simulink model "RflysimIndoorController_r2018b_N6_V8"  (R2018b)
settings: Solver=ode4  StartTime=0.0  StopTime=inf  FixedStep=ts  MaxStep=0.6  RelTol=1e-3
values from neighbouring files (symbols this model uses):
  l_v = 5    [RflyMain.m]    (also in RflyMain_N12_V6.m; RflyMain_N6_V3.m; RflyMain_N6_V4.m; RflyMain_V2.m)
  p_target = [200,10]    [RflyMain.m]    (also in RflyMain_N12_V6.m; RflyMain_N6_V3.m; RflyMain_N6_V4.m; RflyMain_V2.m)
  ra = 0.6    [RflyMain.m]    (also in RflyMain_N12_V6.m; RflyMain_N6_V3.m; RflyMain_N6_V4.m; RflyMain_V2.m)
  rs = 0.25    [RflyMain.m]    (also in RflyMain_N12_V6.m; RflyMain_N6_V3.m; RflyMain_N6_V4.m; RflyMain_V2.m)
  rt1 = 0.25    [RflyMain_N6_V4.m]
  rt2 = 1.5    [RflyMain_N6_V4.m]
  ts = [0 0]    [QuadModel2D.m]    (also in RflyMain.m = 0.01; RflyMain_N12_V6.m = 0.05; RflyMain_N6_V3.m = 0.05; RflyMain_N6_V4.m = 0.05)
  v_max = 2    [RflyMain.m]    (also in RflyMain_N12_V6.m = 3; RflyMain_N6_V3.m = 3; RflyMain_N6_V4.m = 3; RflyMain_V2.m = 3)
undefined symbols (not defined in the file or in its folder): Twist
libraries: robotlib x48, aerolibanimutils x1
settings Model: Creator=51078  LastModifiedBy=root
settings OptimizationCC: EnhancedBackFolding=on  PassReuseOutputArgsAs=Individual arguments  ZeroExternalMemoryAtStartup=off  ZeroInternalMemoryAtStartup=off  MaxStackSize=64  OptimizeBlockOrder=speed  DifferentSizesBufferReuse=on  OptimizationCustomize=off
settings DebuggingCC: ParameterTunabilityLossMsg=error
settings HardwareCC: ProdBitPerPointer=32  ProdBitPerSizeT=32  ProdBitPerPtrDiffT=32  ProdLargestAtomicFloat=None  ProdIntDivRoundTo=Undefined  ProdEndianess=Unspecified  ProdWordSize=32  ProdHWDeviceType=Generic->Unspecified (assume 32-bit Generic)
settings SFSimCC: SimUseLocalCustomCode=off  MATLABDynamicMemAlloc=off
settings RTWCC: SystemTargetFile=ert.tlc  HardwareBoard=Robot Operating System (ROS)  TLCOptions="-aInlineSetEventsForThisBaseRateFcn=TLC_FALSE -aSuppressMultiTaskScheduler=TLC_FALSE  -aRateBasedStepFcn=0"  TemplateMakefile=ert_default_tmf  RTWUseLocalCustomCode=off  Toolchain=Catkin  TargetLang=C++
settings CodeAppCC: ForceParamTrailComments=on  IgnoreCustomStorageClasses=off  OperatorAnnotations=on  SimulinkDataObjDesc=on  SFDataObjDesc=on  InsertBlockDesc=on
settings ERTTargetCC: SupportVariableSizeSignals=on

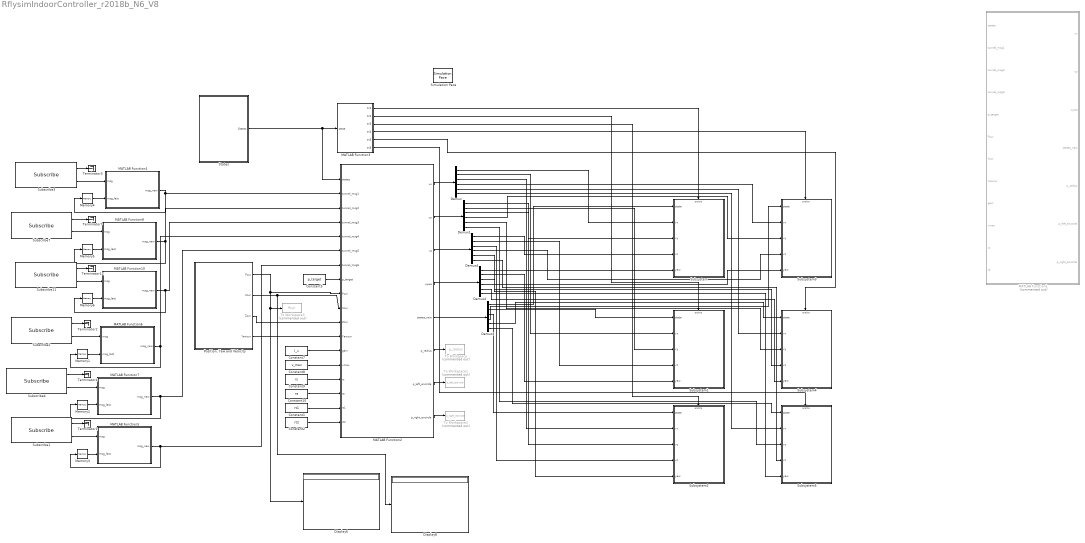
== system RflysimIndoorController_r2018b_N6_V8 ==
  Constant1 : Constant  Value=rt1
  Constant10 : Constant  Value=ra
  Constant2 : Constant  Value=rt2
  Constant5 : Constant  Value=p_target
  Constant7 : Constant  Value=l_v
  Constant8 : Constant  Value=v_max
  Constant9 : Constant  Value=rs
  Demux{,1..4} (5 alike) : Demux  Outputs=6
  Display6 : Display
  Display8 : Display
  MATLAB Function1 : MATLAB Function  Commented=on  TreatAsAtomicUnit=on
  MATLAB Function10 : MATLAB Function  TreatAsAtomicUnit=on
  MATLAB Function2 : MATLAB Function  TreatAsAtomicUnit=on
  MATLAB Function3 : MATLAB Function  TreatAsAtomicUnit=on
  MATLAB Function4 : MATLAB Function  TreatAsAtomicUnit=on
  MATLAB Function5 : MATLAB Function  TreatAsAtomicUnit=on
  MATLAB Function6 : MATLAB Function  TreatAsAtomicUnit=on
  MATLAB Function7 : MATLAB Function  TreatAsAtomicUnit=on
  MATLAB Function8 : MATLAB Function  TreatAsAtomicUnit=on
  Memory{1..6} (6 alike) : Memory
  "Position, Yaw and Velocity" : Subsystem
  Simulation Pace : aerolibanimutils/Simulation Pace  SimulationPace=1  SleepMode=MATLAB Thread  OutputPaceError=off  SampleTime=ts
  States : Subsystem
  Subscribe1 : robotlib/Subscribe  topicSource=Specify your own  topic=/drone_6/decision_info  messageType=swarm_msgs/Pipeline  sampleTime=-1  messageQueueLength=1
  Subscribe11 : robotlib/Subscribe  topicSource=Select from ROS network  topic=/drone_3/decision_info  messageType=swarm_msgs/Pipeline  sampleTime=-1  messageQueueLength=1
  Subscribe2 : robotlib/Subscribe  topicSource=Specify your own  topic=/drone_4/decision_info  messageType=swarm_msgs/Pipeline  sampleTime=-1  messageQueueLength=1
  Subscribe3 : robotlib/Subscribe  topicSource=Select from ROS network  topic=/drone_1/decision_info  messageType=swarm_msgs/Pipeline  sampleTime=-1  messageQueueLength=1
  Subscribe4 : robotlib/Subscribe  topicSource=Specify your own  topic=/drone_5/decision_info  messageType=swarm_msgs/Pipeline  sampleTime=-1  messageQueueLength=1
  Subscribe7 : robotlib/Subscribe  topicSource=Select from ROS network  topic=/drone_2/decision_info  messageType=swarm_msgs/Pipeline  sampleTime=-1  messageQueueLength=1
  Subsystem : Subsystem
  Subsystem1 : Subsystem
  Subsystem2 : Subsystem
  Subsystem3 : Subsystem
  Subsystem4 : Subsystem
  Subsystem5 : Subsystem
  Terminator{1..4,7,11} (6 alike) : Terminator
  To Workspace : ToWorkspace  Commented=on  VariableName=p_radius  SaveFormat=Timeseries  SampleTime=-1
  To Workspace1 : ToWorkspace  Commented=on  VariableName=p_left_encircle  SaveFormat=Timeseries  SampleTime=-1
  To Workspace2 : ToWorkspace  Commented=on  VariableName=p_right_encircle  SaveFormat=Timeseries  SampleTime=-1
  To Workspace3 : ToWorkspace  Commented=on  VariableName=Pcur  SaveFormat=Timeseries  SampleTime=-1
  wires:
  Constant9/1 -> MATLAB Function2/15(rs)
  MATLAB Function2/4(uyaw) -> Demux2/1
  Constant5/1 -> MATLAB Function2/8(p_target)
  Constant7/1 -> MATLAB Function2/13(gain)
  Constant10/1 -> MATLAB Function2/16(ra)
  MATLAB Function2/1(ux) -> Demux/1
  Constant8/1 -> MATLAB Function2/14(vmax)
  MATLAB Function2/5(states_new) -> Demux3/1
  MATLAB Function2/2(uy) -> Demux1/1
  Subscribe3/1 -> Terminator3/1
  MATLAB Function4/1(msg_new) -> Memory4/1, MATLAB Function2/2(tunnel_msg1)
  Subscribe3/2 -> MATLAB Function4/1(msg)
  Memory4/1 -> MATLAB Function4/2(msg_last)
  MATLAB Function2/6(p_radius) -> To Workspace/1
  MATLAB Function2/7(p_left_encircle) -> To Workspace1/1
  MATLAB Function2/8(p_right_encircle) -> To Workspace2/1
  Subscribe7/1 -> Terminator7/1
  Subscribe7/2 -> MATLAB Function8/1(msg)
  Memory5/1 -> MATLAB Function8/2(msg_last)
  MATLAB Function8/1(msg_new) -> MATLAB Function2/3(tunnel_msg2), Memory5/1
  Memory6/1 -> MATLAB Function10/2(msg_last)
  Subscribe11/1 -> Terminator11/1
  Subscribe11/2 -> MATLAB Function10/1(msg)
  MATLAB Function10/1(msg_new) -> Memory6/1, MATLAB Function2/4(tunnel_msg3)
  Demux/1 -> Subsystem/2(vx)
  Demux/2 -> Subsystem1/2(vx)
  Demux/3 -> Subsystem2/2(vx)
  Demux1/1 -> Subsystem/3(vy)
  Demux1/2 -> Subsystem1/3(vy)
  Demux1/3 -> Subsystem2/3(vy)
  Demux2/1 -> Subsystem/5(yaw)
  Demux2/2 -> Subsystem1/5(yaw)
  Demux2/3 -> Subsystem2/5(yaw)
  Demux3/1 -> Subsystem/1(state)
  Demux3/2 -> Subsystem1/1(state)
  Demux3/3 -> Subsystem2/1(state)
  MATLAB Function3/1(tri1) -> Subsystem/Enable
  MATLAB Function3/2(tri2) -> Subsystem1/Enable
  MATLAB Function3/3(tri3) -> Subsystem2/Enable
  States/1(States) -> MATLAB Function2/1(states), MATLAB Function3/1(state)
  "Position, Yaw and Velocity"/2(Vcur) -> Display8/1, MATLAB Function2/10(Vcur)
  "Position, Yaw and Velocity"/1(Pcur) -> To Workspace3/1, Display6/1, MATLAB Function2/9(Pcur)
  "Position, Yaw and Velocity"/4(Yawcur) -> MATLAB Function2/12(Yawcur)
  "Position, Yaw and Velocity"/3(Zcur) -> MATLAB Function2/11(Zcur)
  MATLAB Function2/3(uz) -> Demux4/1
  Demux4/1 -> Subsystem/4(vz)
  Demux4/2 -> Subsystem1/4(vz)
  Demux4/3 -> Subsystem2/4(vz)
  Subscribe2/2 -> MATLAB Function6/1(msg)
  Subscribe1/1 -> Terminator1/1
  Subscribe2/1 -> Terminator2/1
  Subscribe4/1 -> Terminator4/1
  Subscribe4/2 -> MATLAB Function7/1(msg)
  Subscribe1/2 -> MATLAB Function5/1(msg)
  Memory1/1 -> MATLAB Function6/2(msg_last)
  MATLAB Function6/1(msg_new) -> Memory1/1, MATLAB Function2/5(tunnel_msg4)
  MATLAB Function5/1(msg_new) -> MATLAB Function2/7(tunnel_msg6), Memory3/1
  MATLAB Function7/1(msg_new) -> MATLAB Function2/6(tunnel_msg5), Memory2/1
  Memory3/1 -> MATLAB Function5/2(msg_last)
  Memory2/1 -> MATLAB Function7/2(msg_last)
  MATLAB Function3/4(tri4) -> Subsystem3/Enable
  MATLAB Function3/5(tri5) -> Subsystem4/Enable
  MATLAB Function3/6(tri6) -> Subsystem5/Enable
  Demux/4 -> Subsystem3/2(vx)
  Demux/5 -> Subsystem4/2(vx)
  Demux/6 -> Subsystem5/2(vx)
  Demux1/4 -> Subsystem3/3(vy)
  Demux1/5 -> Subsystem4/3(vy)
  Demux1/6 -> Subsystem5/3(vy)
  Demux4/4 -> Subsystem3/4(vz)
  Demux4/5 -> Subsystem4/4(vz)
  Demux4/6 -> Subsystem5/4(vz)
  Demux2/4 -> Subsystem3/5(yaw)
  Demux2/5 -> Subsystem4/5(yaw)
  Demux2/6 -> Subsystem5/5(yaw)
  Demux3/4 -> Subsystem3/1(state)
  Demux3/5 -> Subsystem4/1(state)
  Demux3/6 -> Subsystem5/1(state)
  Constant1/1 -> MATLAB Function2/17(rt1)
  Constant2/1 -> MATLAB Function2/18(rt2)

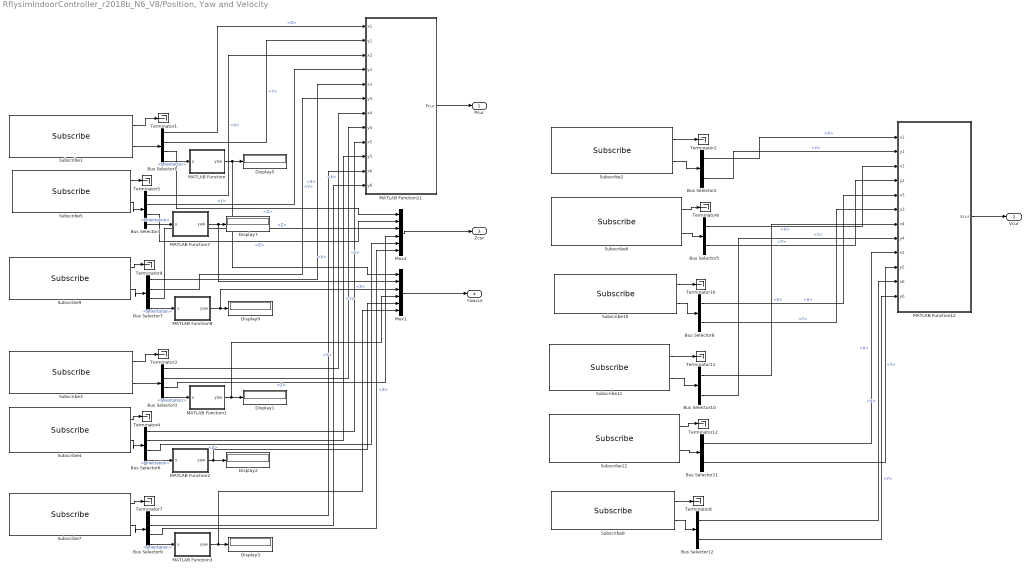
== system RflysimIndoorController_r2018b_N6_V8/Position, Yaw and Velocity ==
  Bus Selector{1,3..4,6..7,9} (6 alike) : BusSelector  OutputSignals=Pose.Position.X,Pose.Position.Y,Pose.Position.Z,Pose.Orientation
  Bus Selector{2,5,8,10..12} (6 alike) : BusSelector  OutputSignals=Twist.Linear.X,Twist.Linear.Y
  Display{1..3,5,7,9} (6 alike) : Display
  MATLAB Function : MATLAB Function  TreatAsAtomicUnit=on
  MATLAB Function1 : MATLAB Function  TreatAsAtomicUnit=on
  MATLAB Function11 : MATLAB Function  TreatAsAtomicUnit=on
  MATLAB Function12 : MATLAB Function  TreatAsAtomicUnit=on
  MATLAB Function2 : MATLAB Function  TreatAsAtomicUnit=on
  MATLAB Function3 : MATLAB Function  TreatAsAtomicUnit=on
  MATLAB Function7 : MATLAB Function  TreatAsAtomicUnit=on
  MATLAB Function9 : MATLAB Function  TreatAsAtomicUnit=on
  Mux1 : Mux  Inputs=6
  Mux2 : Mux  Inputs=6
  Subscribe1 : robotlib/Subscribe  topicSource=Select from ROS network  topic=/drone_1/mavros/local_position/pose_cor  messageType=geometry_msgs/PoseStamped  sampleTime=-1  messageQueueLength=1
  Subscribe10 : robotlib/Subscribe  topicSource=Select from ROS network  topic=/drone_3/mavros/local_position/velocity_local  messageType=geometry_msgs/TwistStamped  sampleTime=-1  messageQueueLength=1
  Subscribe11 : robotlib/Subscribe  topicSource=Specify your own  topic=/drone_4/mavros/local_position/velocity_local  messageType=geometry_msgs/TwistStamped  sampleTime=-1  messageQueueLength=1
  Subscribe12 : robotlib/Subscribe  topicSource=Specify your own  topic=/drone_5/mavros/local_position/velocity_local  messageType=geometry_msgs/TwistStamped  sampleTime=-1  messageQueueLength=1
  Subscribe2 : robotlib/Subscribe  topicSource=Select from ROS network  topic=/drone_1/mavros/local_position/velocity_local  messageType=geometry_msgs/TwistStamped  sampleTime=-1  messageQueueLength=1
  Subscribe3 : robotlib/Subscribe  topicSource=Specify your own  topic=/drone_4/mavros/local_position/pose_cor  messageType=geometry_msgs/PoseStamped  sampleTime=-1  messageQueueLength=1
  Subscribe4 : robotlib/Subscribe  topicSource=Specify your own  topic=/drone_5/mavros/local_position/pose_cor  messageType=geometry_msgs/PoseStamped  sampleTime=-1  messageQueueLength=1
  Subscribe5 : robotlib/Subscribe  topicSource=Select from ROS network  topic=/drone_2/mavros/local_position/pose_cor  messageType=geometry_msgs/PoseStamped  sampleTime=-1  messageQueueLength=1
  Subscribe6 : robotlib/Subscribe  topicSource=Select from ROS network  topic=/drone_2/mavros/local_position/velocity_local  messageType=geometry_msgs/TwistStamped  sampleTime=-1  messageQueueLength=1
  Subscribe7 : robotlib/Subscribe  topicSource=Specify your own  topic=/drone_6/mavros/local_position/pose_cor  messageType=geometry_msgs/PoseStamped  sampleTime=-1  messageQueueLength=1
  Subscribe8 : robotlib/Subscribe  topicSource=Specify your own  topic=/drone_6/mavros/local_position/velocity_local  messageType=geometry_msgs/TwistStamped  sampleTime=-1  messageQueueLength=1
  Subscribe9 : robotlib/Subscribe  topicSource=Select from ROS network  topic=/drone_3/mavros/local_position/pose_cor  messageType=geometry_msgs/PoseStamped  sampleTime=-1  messageQueueLength=1
  Terminator{1..12} (12 alike) : Terminator
  Pcur : Outport
  Vcur : Outport  Port=2
  Zcur : Outport  Port=3
  Yawcur : Outport  Port=4
  wires:
  Subscribe1/1 -> Terminator1/1
  Mux1/1 -> Yawcur/1
  Subscribe10/1 -> Terminator10/1
  MATLAB Function/1(yaw) -> Mux1/1, Display5/1
  Subscribe9/2 -> Bus Selector7/1
  Bus Selector7/3 -> Mux2/3  "<Z>"
  Bus Selector4/3 -> Mux2/2  "<Z>"
  Subscribe5/1 -> Terminator5/1
  Subscribe6/2 -> Bus Selector5/1
  Subscribe9/1 -> Terminator9/1
  Subscribe10/2 -> Bus Selector8/1
  Bus Selector2/2 -> MATLAB Function12/2(y1)  "<Y>"
  Bus Selector4/1 -> MATLAB Function11/3(x2)  "<X>"
  Bus Selector1/1 -> MATLAB Function11/1(x1)  "<X>"
  Subscribe2/1 -> Terminator2/1
  Subscribe2/2 -> Bus Selector2/1
  Bus Selector5/2 -> MATLAB Function12/4(y2)  "<Y>"
  MATLAB Function12/1(Vcur) -> Vcur/1
  Bus Selector8/1 -> MATLAB Function12/5(x3)  "<X>"
  Bus Selector5/1 -> MATLAB Function12/3(x2)  "<X>"
  Subscribe1/2 -> Bus Selector1/1
  Bus Selector7/2 -> MATLAB Function11/6(y3)  "<Y>"
  Bus Selector8/2 -> MATLAB Function12/6(y3)  "<Y>"
  Bus Selector4/2 -> MATLAB Function11/4(y2)  "<Y>"
  Subscribe6/1 -> Terminator6/1
  Bus Selector7/1 -> MATLAB Function11/5(x3)  "<X>"
  Bus Selector4/4 -> MATLAB Function7/1(u)  "<Orientation>"
  Bus Selector1/4 -> MATLAB Function/1(u)  "<Orientation>"
  MATLAB Function11/1(Pcur) -> Pcur/1
  Bus Selector7/4 -> MATLAB Function9/1(u)  "<Orientation>"
  MATLAB Function7/1(yaw) -> Mux1/2, Display7/1
  Mux2/1 -> Zcur/1
  Bus Selector2/1 -> MATLAB Function12/1(x1)  "<X>"
  MATLAB Function9/1(yaw) -> Mux1/3, Display9/1
  Bus Selector1/2 -> MATLAB Function11/2(y1)  "<Y>"
  Subscribe5/2 -> Bus Selector4/1
  Bus Selector1/3 -> Mux2/1  "<Z>"
  Subscribe4/1 -> Terminator4/1
  Bus Selector3/4 -> MATLAB Function1/1(u)  "<Orientation>"
  Bus Selector9/4 -> MATLAB Function3/1(u)  "<Orientation>"
  Subscribe7/1 -> Terminator7/1
  MATLAB Function3/1(yaw) -> Mux1/6, Display3/1
  Subscribe3/1 -> Terminator3/1
  MATLAB Function2/1(yaw) -> Mux1/5, Display2/1
  Bus Selector6/4 -> MATLAB Function2/1(u)  "<Orientation>"
  MATLAB Function1/1(yaw) -> Mux1/4, Display1/1
  Subscribe7/2 -> Bus Selector9/1
  Subscribe4/2 -> Bus Selector6/1
  Subscribe3/2 -> Bus Selector3/1
  Bus Selector3/1 -> MATLAB Function11/7(x4)  "<X>"
  Bus Selector3/2 -> MATLAB Function11/8(y4)  "<Y>"
  Bus Selector6/1 -> MATLAB Function11/9(x5)  "<X>"
  Bus Selector6/2 -> MATLAB Function11/10(y5)  "<Y>"
  Bus Selector9/1 -> MATLAB Function11/11(x6)  "<X>"
  Bus Selector9/2 -> MATLAB Function11/12(y6)  "<Y>"
  Bus Selector3/3 -> Mux2/4  "<Z>"
  Bus Selector6/3 -> Mux2/5  "<Z>"
  Bus Selector9/3 -> Mux2/6  "<Z>"
  Subscribe12/1 -> Terminator12/1
  Subscribe8/2 -> Bus Selector12/1
  Subscribe12/2 -> Bus Selector11/1
  Subscribe11/2 -> Bus Selector10/1
  Subscribe11/1 -> Terminator11/1
  Subscribe8/1 -> Terminator8/1
  Bus Selector10/1 -> MATLAB Function12/7(x4)  "<X>"
  Bus Selector10/2 -> MATLAB Function12/8(y4)  "<Y>"
  Bus Selector11/1 -> MATLAB Function12/9(x5)  "<X>"
  Bus Selector11/2 -> MATLAB Function12/10(y5)  "<Y>"
  Bus Selector12/1 -> MATLAB Function12/11(x6)  "<X>"
  Bus Selector12/2 -> MATLAB Function12/12(y6)  "<Y>"

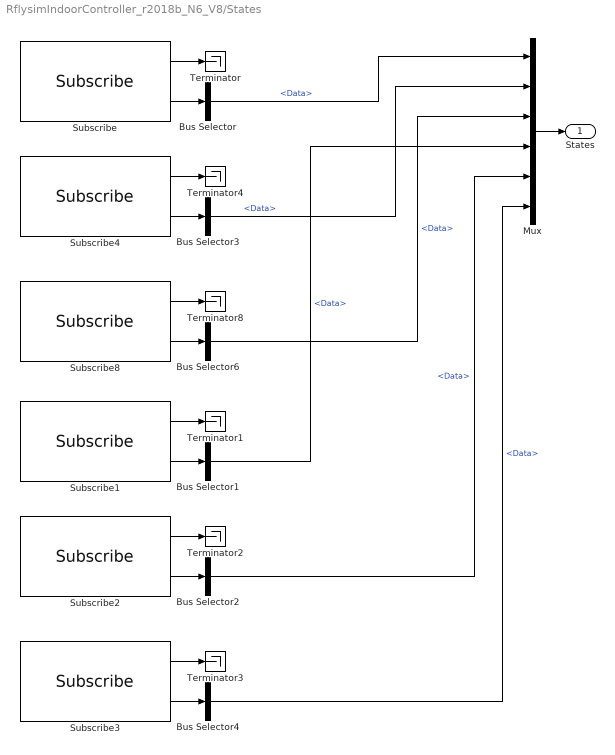
== system RflysimIndoorController_r2018b_N6_V8/States ==
  Bus Selector{,1..4,6} (6 alike) : BusSelector  OutputSignals=Data
  Mux : Mux  Inputs=6
  Subscribe : robotlib/Subscribe  topicSource=Select from ROS network  topic=/drone_1/state  messageType=std_msgs/UInt64  sampleTime=-1  messageQueueLength=1
  Subscribe1 : robotlib/Subscribe  topicSource=Specify your own  topic=/drone_4/state  messageType=std_msgs/UInt64  sampleTime=-1  messageQueueLength=1
  Subscribe2 : robotlib/Subscribe  topicSource=Specify your own  topic=/drone_5/state  messageType=std_msgs/UInt64  sampleTime=-1  messageQueueLength=1
  Subscribe3 : robotlib/Subscribe  topicSource=Specify your own  topic=/drone_6/state  messageType=std_msgs/UInt64  sampleTime=-1  messageQueueLength=1
  Subscribe4 : robotlib/Subscribe  topicSource=Select from ROS network  topic=/drone_2/state  messageType=std_msgs/UInt64  sampleTime=-1  messageQueueLength=1
  Subscribe8 : robotlib/Subscribe  topicSource=Select from ROS network  topic=/drone_3/state  messageType=std_msgs/UInt64  sampleTime=-1  messageQueueLength=1
  Terminator{,1..4,8} (6 alike) : Terminator
  States : Outport
  wires:
  Bus Selector3/1 -> Mux/2  "<Data>"
  Subscribe4/2 -> Bus Selector3/1
  Subscribe/2 -> Bus Selector/1
  Subscribe4/1 -> Terminator4/1
  Bus Selector6/1 -> Mux/3  "<Data>"
  Subscribe8/2 -> Bus Selector6/1
  Bus Selector/1 -> Mux/1  "<Data>"
  Subscribe/1 -> Terminator/1
  Subscribe8/1 -> Terminator8/1
  Mux/1 -> States/1
  Subscribe3/1 -> Terminator3/1
  Subscribe3/2 -> Bus Selector4/1
  Bus Selector4/1 -> Mux/6  "<Data>"
  Subscribe1/1 -> Terminator1/1
  Bus Selector1/1 -> Mux/4  "<Data>"
  Bus Selector2/1 -> Mux/5  "<Data>"
  Subscribe1/2 -> Bus Selector1/1
  Subscribe2/1 -> Terminator2/1
  Subscribe2/2 -> Bus Selector2/1

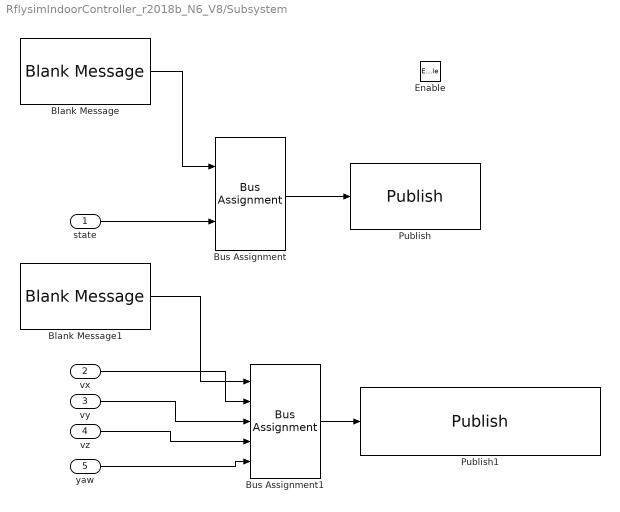
== system RflysimIndoorController_r2018b_N6_V8/Subsystem ==
  state : Inport
  vx : Inport  Port=2
  vy : Inport  Port=3
  vz : Inport  Port=4
  yaw : Inport  Port=5
  Enable : EnablePort
  Blank Message : robotlib/Blank Message  messageClass=Message  entityType=std_msgs/UInt64  messageType=std_msgs/UInt64  SampleTime=inf
  Blank Message1 : robotlib/Blank Message  messageClass=Message  entityType=geometry_msgs/TwistStamped  messageType=geometry_msgs/TwistStamped  SampleTime=inf
  Bus Assignment : BusAssignment  AssignedSignals=Data
  Bus Assignment1 : BusAssignment  AssignedSignals=Twist.Linear.X,Twist.Linear.Y,Twist.Linear.Z,Twist.Angular.Z
  Publish : robotlib/Publish  topicSource=Select from ROS network  topic=/drone_1/state  messageType=std_msgs/UInt64  messageQueueLength=1
  Publish1 : robotlib/Publish  topicSource=Select from ROS network  topic=/drone_1/mavros/setpoint_velocity/cmd_vel  messageType=geometry_msgs/TwistStamped  messageQueueLength=1
  wires:
  Blank Message/1 -> Bus Assignment/1
  state/1 -> Bus Assignment/2
  Bus Assignment/1 -> Publish/1
  Bus Assignment1/1 -> Publish1/1
  Blank Message1/1 -> Bus Assignment1/1
  vx/1 -> Bus Assignment1/2
  vy/1 -> Bus Assignment1/3
  yaw/1 -> Bus Assignment1/5
  vz/1 -> Bus Assignment1/4

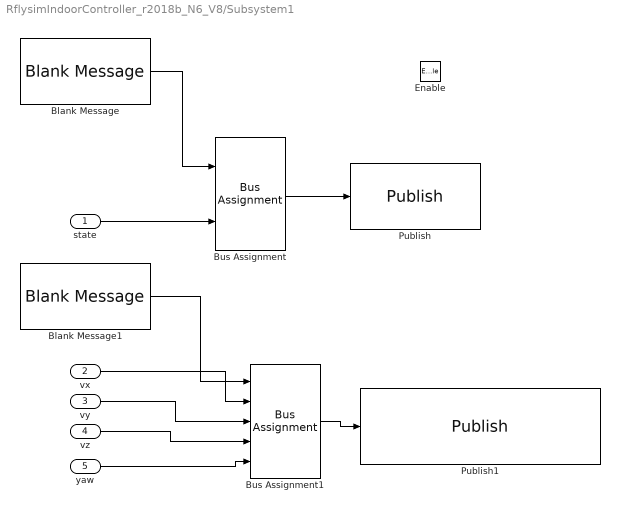
== system RflysimIndoorController_r2018b_N6_V8/Subsystem1 ==
  state : Inport
  vx : Inport  Port=2
  vy : Inport  Port=3
  vz : Inport  Port=4
  yaw : Inport  Port=5
  Enable : EnablePort
  Blank Message : robotlib/Blank Message  messageClass=Message  entityType=std_msgs/UInt64  messageType=std_msgs/UInt64  SampleTime=inf
  Blank Message1 : robotlib/Blank Message  messageClass=Message  entityType=geometry_msgs/TwistStamped  messageType=geometry_msgs/TwistStamped  SampleTime=inf
  Bus Assignment : BusAssignment  AssignedSignals=Data
  Bus Assignment1 : BusAssignment  AssignedSignals=Twist.Linear.X,Twist.Linear.Y,Twist.Linear.Z,Twist.Angular.Z
  Publish : robotlib/Publish  topicSource=Select from ROS network  topic=/drone_2/state  messageType=std_msgs/UInt64  messageQueueLength=1
  Publish1 : robotlib/Publish  topicSource=Select from ROS network  topic=/drone_2/mavros/setpoint_velocity/cmd_vel  messageType=geometry_msgs/TwistStamped  messageQueueLength=1
  wires:
  Blank Message/1 -> Bus Assignment/1
  state/1 -> Bus Assignment/2
  Bus Assignment/1 -> Publish/1
  Bus Assignment1/1 -> Publish1/1
  Blank Message1/1 -> Bus Assignment1/1
  vx/1 -> Bus Assignment1/2
  vy/1 -> Bus Assignment1/3
  yaw/1 -> Bus Assignment1/5
  vz/1 -> Bus Assignment1/4

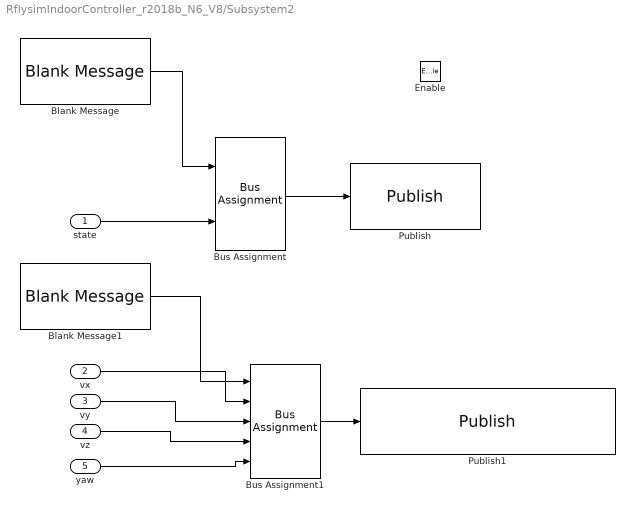
== system RflysimIndoorController_r2018b_N6_V8/Subsystem2 ==
  state : Inport
  vx : Inport  Port=2
  vy : Inport  Port=3
  vz : Inport  Port=4
  yaw : Inport  Port=5
  Enable : EnablePort
  Blank Message : robotlib/Blank Message  messageClass=Message  entityType=std_msgs/UInt64  messageType=std_msgs/UInt64  SampleTime=inf
  Blank Message1 : robotlib/Blank Message  messageClass=Message  entityType=geometry_msgs/TwistStamped  messageType=geometry_msgs/TwistStamped  SampleTime=inf
  Bus Assignment : BusAssignment  AssignedSignals=Data
  Bus Assignment1 : BusAssignment  AssignedSignals=Twist.Linear.X,Twist.Linear.Y,Twist.Linear.Z,Twist.Angular.Z
  Publish : robotlib/Publish  topicSource=Select from ROS network  topic=/drone_3/state  messageType=std_msgs/UInt64  messageQueueLength=1
  Publish1 : robotlib/Publish  topicSource=Select from ROS network  topic=/drone_3/mavros/setpoint_velocity/cmd_vel  messageType=geometry_msgs/TwistStamped  messageQueueLength=1
  wires:
  Blank Message/1 -> Bus Assignment/1
  state/1 -> Bus Assignment/2
  Bus Assignment/1 -> Publish/1
  Bus Assignment1/1 -> Publish1/1
  Blank Message1/1 -> Bus Assignment1/1
  vx/1 -> Bus Assignment1/2
  vy/1 -> Bus Assignment1/3
  yaw/1 -> Bus Assignment1/5
  vz/1 -> Bus Assignment1/4

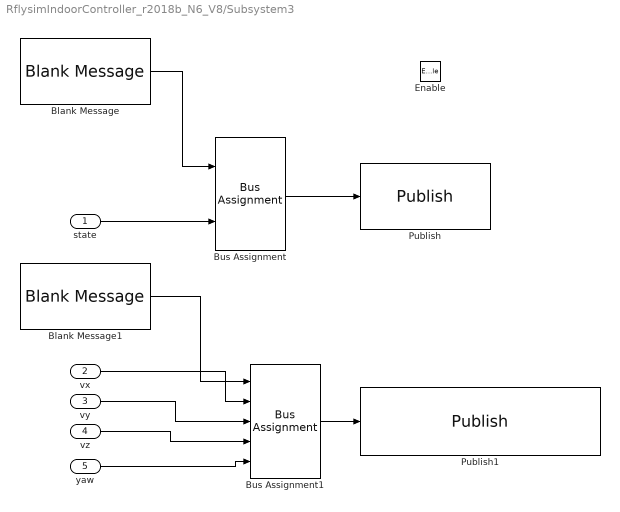
== system RflysimIndoorController_r2018b_N6_V8/Subsystem3 ==
  state : Inport
  vx : Inport  Port=2
  vy : Inport  Port=3
  vz : Inport  Port=4
  yaw : Inport  Port=5
  Enable : EnablePort
  Blank Message : robotlib/Blank Message  messageClass=Message  entityType=std_msgs/UInt64  messageType=std_msgs/UInt64  SampleTime=inf
  Blank Message1 : robotlib/Blank Message  messageClass=Message  entityType=geometry_msgs/TwistStamped  messageType=geometry_msgs/TwistStamped  SampleTime=inf
  Bus Assignment : BusAssignment  AssignedSignals=Data
  Bus Assignment1 : BusAssignment  AssignedSignals=Twist.Linear.X,Twist.Linear.Y,Twist.Linear.Z,Twist.Angular.Z
  Publish : robotlib/Publish  topicSource=Specify your own  topic=/drone_4/state  messageType=std_msgs/UInt64  messageQueueLength=1
  Publish1 : robotlib/Publish  topicSource=Specify your own  topic=/drone_4/mavros/setpoint_velocity/cmd_vel  messageType=geometry_msgs/TwistStamped  messageQueueLength=1
  wires:
  Blank Message/1 -> Bus Assignment/1
  state/1 -> Bus Assignment/2
  Bus Assignment/1 -> Publish/1
  Bus Assignment1/1 -> Publish1/1
  Blank Message1/1 -> Bus Assignment1/1
  vx/1 -> Bus Assignment1/2
  vy/1 -> Bus Assignment1/3
  yaw/1 -> Bus Assignment1/5
  vz/1 -> Bus Assignment1/4

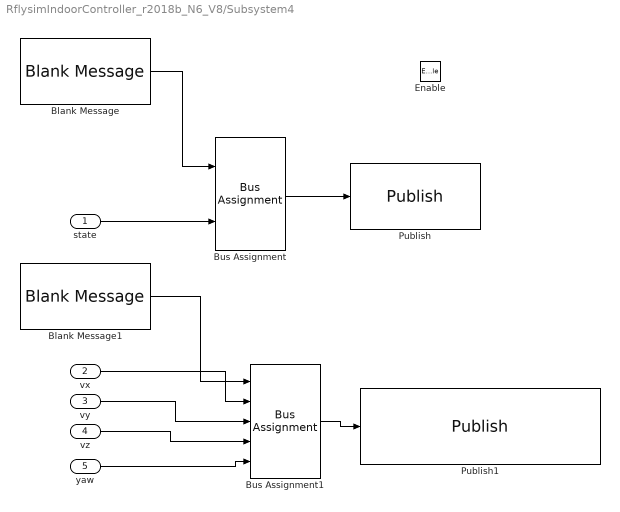
== system RflysimIndoorController_r2018b_N6_V8/Subsystem4 ==
  state : Inport
  vx : Inport  Port=2
  vy : Inport  Port=3
  vz : Inport  Port=4
  yaw : Inport  Port=5
  Enable : EnablePort
  Blank Message : robotlib/Blank Message  messageClass=Message  entityType=std_msgs/UInt64  messageType=std_msgs/UInt64  SampleTime=inf
  Blank Message1 : robotlib/Blank Message  messageClass=Message  entityType=geometry_msgs/TwistStamped  messageType=geometry_msgs/TwistStamped  SampleTime=inf
  Bus Assignment : BusAssignment  AssignedSignals=Data
  Bus Assignment1 : BusAssignment  AssignedSignals=Twist.Linear.X,Twist.Linear.Y,Twist.Linear.Z,Twist.Angular.Z
  Publish : robotlib/Publish  topicSource=Specify your own  topic=/drone_5/state  messageType=std_msgs/UInt64  messageQueueLength=1
  Publish1 : robotlib/Publish  topicSource=Specify your own  topic=/drone_5/mavros/setpoint_velocity/cmd_vel  messageType=geometry_msgs/TwistStamped  messageQueueLength=1
  wires:
  Blank Message/1 -> Bus Assignment/1
  state/1 -> Bus Assignment/2
  Bus Assignment/1 -> Publish/1
  Bus Assignment1/1 -> Publish1/1
  Blank Message1/1 -> Bus Assignment1/1
  vx/1 -> Bus Assignment1/2
  vy/1 -> Bus Assignment1/3
  yaw/1 -> Bus Assignment1/5
  vz/1 -> Bus Assignment1/4

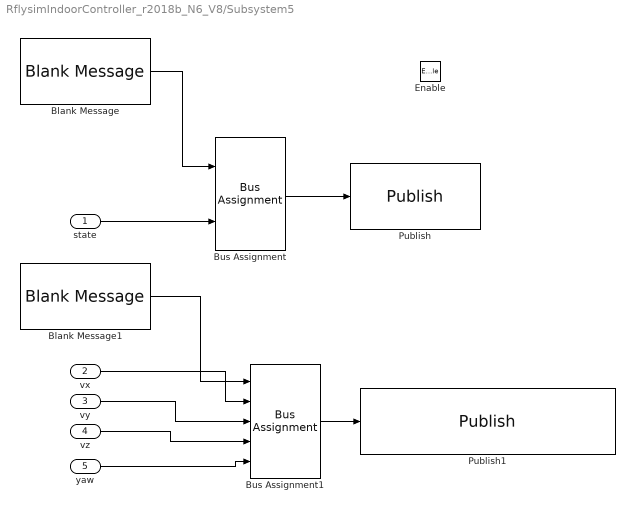
== system RflysimIndoorController_r2018b_N6_V8/Subsystem5 ==
  state : Inport
  vx : Inport  Port=2
  vy : Inport  Port=3
  vz : Inport  Port=4
  yaw : Inport  Port=5
  Enable : EnablePort
  Blank Message : robotlib/Blank Message  messageClass=Message  entityType=std_msgs/UInt64  messageType=std_msgs/UInt64  SampleTime=inf
  Blank Message1 : robotlib/Blank Message  messageClass=Message  entityType=geometry_msgs/TwistStamped  messageType=geometry_msgs/TwistStamped  SampleTime=inf
  Bus Assignment : BusAssignment  AssignedSignals=Data
  Bus Assignment1 : BusAssignment  AssignedSignals=Twist.Linear.X,Twist.Linear.Y,Twist.Linear.Z,Twist.Angular.Z
  Publish : robotlib/Publish  topicSource=Specify your own  topic=/drone_6/state  messageType=std_msgs/UInt64  messageQueueLength=1
  Publish1 : robotlib/Publish  topicSource=Specify your own  topic=/drone_6/mavros/setpoint_velocity/cmd_vel  messageType=geometry_msgs/TwistStamped  messageQueueLength=1
  wires:
  Blank Message/1 -> Bus Assignment/1
  state/1 -> Bus Assignment/2
  Bus Assignment/1 -> Publish/1
  Bus Assignment1/1 -> Publish1/1
  Blank Message1/1 -> Bus Assignment1/1
  vx/1 -> Bus Assignment1/2
  vy/1 -> Bus Assignment1/3
  yaw/1 -> Bus Assignment1/5
  vz/1 -> Bus Assignment1/4

== matlab function RflysimIndoorController_r2018b_N6_V8/MATLAB Function1 ==
  data: states input; tunnel_msg1 input; tunnel_msg2 input; tunnel_msg3 input; ux output; uy output; p_target input; Pcur input; Vcur input; Yawcur input; gain input; vmax input; uyaw output; rs input; ra input; states_new output; p_radius output; p_left_encircle output; p_right_encircle output
function [ux,uy,uyaw,states_new,p_radius,p_left_encircle,p_right_encircle]  = mytunnel(states,tunnel_msg1,tunnel_msg2,tunnel_msg3,p_target,Pcur,Vcur,Yawcur,gain,vmax,rs,ra)
p_target=p_target';

N=3;
ux=zeros(N,1);
uy=zeros(N,1);
uyaw=zeros(N,1);
states_new=zeros(N,1);
tunnel_msg=tunnel_msg1;    
for j=1:N
    
    left_x=zeros(10,1);
    left_y=zeros(10,1);
    right_x=zeros(10,1);
    right_y=zeros(10,1);
    middle_x=zeros(10,1);
    middle_y=zeros(10,1);
    if j==1
        tunnel_msg=tunnel_msg1;
    elseif j==2
        tunnel_msg=tunnel_msg2;
    elseif j==3
        tunnel_msg=tunnel_msg3;
    end
    
    tunnel_type = tunnel_msg.Pipetype.Data;
    point_num=tunnel_msg.Units_SL_Info.CurrentLength;
    
    for k=1:point_num
        left_x(k,1) = tunnel_msg.Units(k).Left.X;
        left_y(k,1) = tunnel_msg.Units(k).Left.Y;
        
        right_x(k,1) = tunnel_msg.Units(k).Right.X;
        right_y(k,1) = tunnel_msg.Units(k).Right.Y;
        
        middle_x(k,1) = tunnel_msg.Units(k).Middle.X;
        middle_y(k,1) = tunnel_msg.Units(k).Middle.Y;
    end
    
    left_x=left_x(1:point_num,1);
    left_y=left_y(1:point_num,1);
    right_x=right_x(1:point_num,1);
    right_y=right_y(1:point_num,1);
    middle_x=middle_x(1:point_num,1);
    middle_y=middle_y(1:point_num,1);

    inter_num = 100;
    p_radius=zeros(inter_num,2);
    p_left_encircle=zeros(inter_num,2);
    p_right_encircle=zeros(inter_num,2);
    
    if tunnel_type==10
        k=1:length(middle_x);
        ki=linspace(1,length(middle_x),inter_num); %%%%% 插值的点越多，控制更精确，曲线更光滑，计算更耗时
        p_radius_x=(interp1(k,middle_x,ki,'pchip'))';
        p_radius_y=(interp1(k,middle_y,ki,'pchip'))';
        for i=1:length(p_radius(:,1))
            p_radius(i,1)=p_radius_x(i);
            p_radius(i,2)=p_radius_y(i);
        end
        
        k=1:length(left_x);
        ki=linspace(1,length(left_x),inter_num); %%%%% 插值的点越多，控制更精确，曲线更光滑，计算更耗时
        p_left_encircle_x=(interp1(k,left_x,ki,'pchip'))';
        p_left_encircle_y=(interp1(k,left_y,ki,'pchip'))';
        for i=1:length(p_left_encircle(:,1))
            p_left_encircle(i,1)=p_left_encircle_x(i);
            p_left_encircle(i,2)=p_left_encircle_y(i);
        end
        
        k=1:length(right_x);
        ki=linspace(1,length(right_x),inter_num); %%%%% 插值的点越多，控制更精确，曲线更光滑，计算更耗时
        p_right_encircle_x=(interp1(k,right_x,ki,'pchip'))';
        p_right_encircle_y=(interp1(k,right_y,ki,'pchip'))';
        for i=1:length(p_right_encircle(:,1))
            p_right_encircle(i,1)=p_right_encircle_x(i);
            p_right_encircle(i,2)=p_right_encircle_y(i);
        end
    end


    
    [u_encircle,ux_encircle,uy_encircle,uyaw_encircle,leader_locate,dist_encircle]  = Encirclement2(p_radius,p_left_encircle,p_right_encircle,p_target,Pcur,Vcur,Yawcur,gain,vmax,rs,ra,j);
    
    if states(j)==30
        states_new(j)=30;
        if tunnel_type==10
            ux(j)=ux_encircle;
            uy(j)=uy_encircle;
            uyaw(j)=uyaw_encircle;
            if abs(leader_locate-inter_num)<5
                states_new(j)=20;
            end
        end
    end
end

== matlab function RflysimIndoorController_r2018b_N6_V8/MATLAB Function2 ==
  data: states input; tunnel_msg1 input; tunnel_msg2 input; tunnel_msg3 input; tunnel_msg4 input; tunnel_msg5 input; tunnel_msg6 input; ux output; uy output; uz output; p_target input; Pcur input; Vcur input; Zcur input; Yawcur input; gain input; vmax input; uyaw output; rs input; ra input; states_new output; p_radius output; p_left_encircle output; p_right_encircle output; rt1 input; rt2 input
function [ux,uy,uz,uyaw,states_new,p_radius,p_left_encircle,p_right_encircle]  = mytunnel(states,tunnel_msg1,tunnel_msg2,tunnel_msg3,tunnel_msg4,tunnel_msg5,tunnel_msg6,p_target,Pcur,Vcur,Zcur,Yawcur,gain,vmax,rs,ra,rt1,rt2)
p_target=p_target';

N=6;
ux=zeros(N,1);
uy=zeros(N,1);
uz=zeros(N,1);
uyaw=zeros(N,1);
states_new=zeros(N,1);
tunnel_msg=tunnel_msg1;
height_desire=4;

for j=1:N
    uz(j)=mysatNum((height_desire-Zcur(j))*0.8,-2,2);
    
    left_x=zeros(10,1);
    left_y=zeros(10,1);
    right_x=zeros(10,1);
    right_y=zeros(10,1);
    middle_x=zeros(10,1);
    middle_y=zeros(10,1);
    if j==1
        tunnel_msg=tunnel_msg1;
    elseif j==2
        tunnel_msg=tunnel_msg2;
    elseif j==3
        tunnel_msg=tunnel_msg3;
    elseif j==4
        tunnel_msg=tunnel_msg4;
    elseif j==5
        tunnel_msg=tunnel_msg5;
    elseif j==6
        tunnel_msg=tunnel_msg6;
    end
    tunnel_type = tunnel_msg.Pipetype.Data;
    point_num=tunnel_msg.Units_SL_Info.CurrentLength;
    
    for k=1:point_num
        left_x(k,1) = tunnel_msg.Units(k).Left.X;
        left_y(k,1) = tunnel_msg.Units(k).Left.Y;
        
        right_x(k,1) = tunnel_msg.Units(k).Right.X;
        right_y(k,1) = tunnel_msg.Units(k).Right.Y;
        
        middle_x(k,1) = tunnel_msg.Units(k).Middle.X;
        middle_y(k,1) = tunnel_msg.Units(k).Middle.Y;
    end
    
    left_x=left_x(1:point_num,1);
    left_y=left_y(1:point_num,1);
    right_x=right_x(1:point_num,1);
    right_y=right_y(1:point_num,1);
    middle_x=middle_x(1:point_num,1);
    middle_y=middle_y(1:point_num,1);
    
    inter_num = 500;
    p_radius=zeros(inter_num,2);
    p_left_encircle=zeros(inter_num,2);
    p_right_encircle=zeros(inter_num,2);
    
    if tunnel_type==10
        k=1:length(middle_x);
        ki=linspace(1,length(middle_x),inter_num); %%%%% 插值的点越多，控制更精确，曲线更光滑，计算更耗时
        p_radius_x=(interp1(k,middle_x,ki,'linear'))';
        p_radius_y=(interp1(k,middle_y,ki,'linear'))';
        p_radius(:,1)=p_radius_x;
        p_radius(:,2)=p_radius_y;
        
        k=1:length(left_x);
        ki=linspace(1,length(left_x),inter_num); %%%%% 插值的点越多，控制更精确，曲线更光滑，计算更耗时
        p_left_encircle_x=(interp1(k,left_x,ki,'linear'))';
        p_left_encircle_y=(interp1(k,left_y,ki,'linear'))';

        p_left_encircle(:,1)=p_left_encircle_x;
        p_left_encircle(:,2)=p_left_encircle_y;
        
        k=1:length(right_x);
        ki=linspace(1,length(right_x),inter_num); %%%%% 插值的点越多，控制更精确，曲线更光滑，计算更耗时
        p_right_encircle_x=(interp1(k,right_x,ki,'linear'))';
        p_right_encircle_y=(interp1(k,right_y,ki,'linear'))';
        p_right_encircle(:,1)=p_right_encircle_x;
        p_right_encircle(:,2)=p_right_encircle_y;
    end
    
    
    
    [u_encircle,ux_encircle,uy_encircle,uyaw_encircle,leader_locate,dist_encircle]  = Encirclement4(p_radius,p_left_encircle,p_right_encircle,p_target,Pcur,Vcur,Yawcur,gain,vmax,rs,ra,rt1,rt2,j);
    
    if states(j)==30
        states_new(j)=30;
        if tunnel_type==10
            ux(j)=ux_encircle;
            uy(j)=uy_encircle;
            uyaw(j)=uyaw_encircle;
            if abs(leader_locate-inter_num)<5
                states_new(j)=20;
            end
        end
    end
end

== matlab function RflysimIndoorController_r2018b_N6_V8/Position, Yaw and Velocity/MATLAB Function ==
  data: u input; yaw output
function yaw = fcn(u)
q0=u.W;
q1=u.X;
q2=u.Y;
q3=u.Z;
yaw = atan2(2*(q0*q3+q1*q2), 1-2*(q2*q2+q3*q3));

== matlab function RflysimIndoorController_r2018b_N6_V8/MATLAB Function3 ==
  data: state input; tri1 output; tri2 output; tri3 output; tri4 output; tri5 output; tri6 output
function [tri1,tri2,tri3,tri4,tri5,tri6] = fcn(state)
tri1=0;
tri2=0;
tri3=0;
tri4=0;
tri5=0;
tri6=0;

if state(1)==30
    tri1=1;
end
if state(2)==30
    tri2=1;
end
if state(3)==30
    tri3=1;
end
if state(4)==30
    tri4=1;
end
if state(5)==30
    tri5=1;
end
if state(6)==30
    tri6=1;
end

== matlab function RflysimIndoorController_r2018b_N6_V8/MATLAB Function4 ==
  data: msg input; msg_new output Bus_type; msg_last input
function msg_new = fcn(msg,msg_last)
if msg.Units_SL_Info.CurrentLength==0
    msg_new=msg_last;
else
    msg_new=msg;
end

== matlab function RflysimIndoorController_r2018b_N6_V8/MATLAB Function5 ==
  data: msg input; msg_new output Bus_type; msg_last input
function msg_new = fcn(msg,msg_last)
if msg.Units_SL_Info.CurrentLength==0
    msg_new=msg_last;
else
    msg_new=msg;
end

== matlab function RflysimIndoorController_r2018b_N6_V8/MATLAB Function6 ==
  data: msg input; msg_new output Bus_type; msg_last input
function msg_new = fcn(msg,msg_last)
if msg.Units_SL_Info.CurrentLength==0
    msg_new=msg_last;
else
    msg_new=msg;
end

== matlab function RflysimIndoorController_r2018b_N6_V8/Position, Yaw and Velocity/MATLAB Function7 ==
  data: u input; yaw output
function yaw = fcn(u)
q0=u.W;
q1=u.X;
q2=u.Y;
q3=u.Z;
yaw = atan2(2*(q0*q3+q1*q2), 1-2*(q2*q2+q3*q3));

== matlab function RflysimIndoorController_r2018b_N6_V8/MATLAB Function8 ==
  data: msg input; msg_new output Bus_type; msg_last input
function msg_new = fcn(msg,msg_last)
if msg.Units_SL_Info.CurrentLength==0
    msg_new=msg_last;
else
    msg_new=msg;
end

== matlab function RflysimIndoorController_r2018b_N6_V8/MATLAB Function10 ==
  data: msg input; msg_new output Bus: SL_Bus_RflysimIndoorController_r_Pipeline_xokozg; msg_last input
function msg_new = fcn(msg,msg_last)
if msg.Units_SL_Info.CurrentLength==0
    msg_new=msg_last;
else
    msg_new=msg;
end

== matlab function RflysimIndoorController_r2018b_N6_V8/Position, Yaw and Velocity/MATLAB Function9 ==
  data: u input; yaw output
function yaw = fcn(u)
q0=u.W;
q1=u.X;
q2=u.Y;
q3=u.Z;
yaw = atan2(2*(q0*q3+q1*q2), 1-2*(q2*q2+q3*q3));

== matlab function RflysimIndoorController_r2018b_N6_V8/Position, Yaw and Velocity/MATLAB Function11 ==
  data: x1 input; Pcur output; y1 input; x2 input; y2 input; x3 input; y3 input; x4 input; y4 input; x5 input; y5 input; x6 input; y6 input
function Pcur = fcn(x1,y1,x2,y2,x3,y3,x4,y4,x5,y5,x6,y6)
Pcur=[x1,y1;x2,y2;x3,y3;x4,y4;x5,y5;x6,y6];

== matlab function RflysimIndoorController_r2018b_N6_V8/Position, Yaw and Velocity/MATLAB Function12 ==
  data: x1 input; Vcur output; y1 input; x2 input; y2 input; x3 input; y3 input; x4 input; y4 input; x5 input; y5 input; x6 input; y6 input
function Vcur = fcn(x1,y1,x2,y2,x3,y3,x4,y4,x5,y5,x6,y6)
Vcur=[x1,y1;x2,y2;x3,y3;x4,y4;x5,y5;x6,y6];

== matlab function RflysimIndoorController_r2018b_N6_V8/MATLAB Function7 ==
  data: msg input; msg_new output Bus_type; msg_last input
function msg_new = fcn(msg,msg_last)
if msg.Units_SL_Info.CurrentLength==0
    msg_new=msg_last;
else
    msg_new=msg;
end

== matlab function RflysimIndoorController_r2018b_N6_V8/Position, Yaw and Velocity/MATLAB Function1 ==
  data: u input; yaw output
function yaw = fcn(u)
q0=u.W;
q1=u.X;
q2=u.Y;
q3=u.Z;
yaw = atan2(2*(q0*q3+q1*q2), 1-2*(q2*q2+q3*q3));

== matlab function RflysimIndoorController_r2018b_N6_V8/Position, Yaw and Velocity/MATLAB Function2 ==
  data: u input; yaw output
function yaw = fcn(u)
q0=u.W;
q1=u.X;
q2=u.Y;
q3=u.Z;
yaw = atan2(2*(q0*q3+q1*q2), 1-2*(q2*q2+q3*q3));

== matlab function RflysimIndoorController_r2018b_N6_V8/Position, Yaw and Velocity/MATLAB Function3 ==
  data: u input; yaw output
function yaw = fcn(u)
q0=u.W;
q1=u.X;
q2=u.Y;
q3=u.Z;
yaw = atan2(2*(q0*q3+q1*q2), 1-2*(q2*q2+q3*q3));
